simulink model "three_pole_pi"  (R2025b)
settings: Solver=VariableStepAuto  StartTime=0.0  StopTime=120  RelTol=1e-3
model workspace (MAT data in the model file):
  Ki = 20
  Kp = 250
  b = 50
  m = 1000
  u = 10
values from neighbouring files (symbols this model uses):
  l_eff = 9.8/(omega_n^2)    [Rocky_pendulum_parametization.m]
  omega_n = signal_params.omega_n    [Rocky_pendulum_parametization.m]
undefined symbols (not defined in the file or in its folder): alpha, beta
settings Model: Creator=clee1  LastModifiedBy=ssocol
settings SolverCC: AlgebraicLoopSolver=TrustRegion
settings DebuggingCC: UnconnectedInputMsg=warning  UnconnectedOutputMsg=warning  UnconnectedLineMsg=warning
settings ModelReferenceCC: EnableRefExpFcnMdlSchedulingChecks=on
settings RTWCC: GPUComputeCapability=3.5

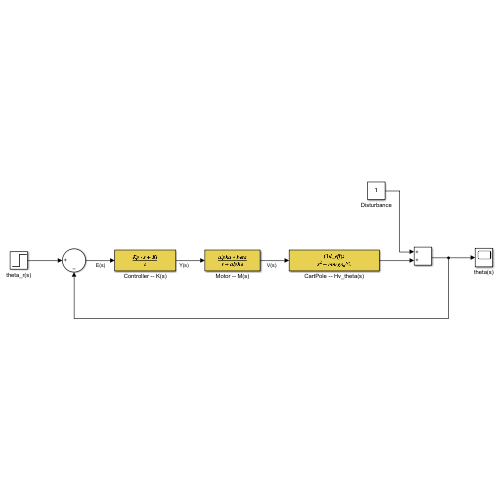
[thumbnail: Simulink's stored preview of the top-level diagram]
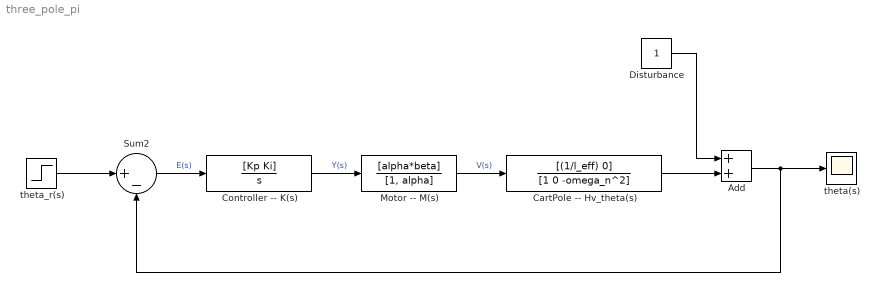
== system three_pole_pi ==
  Add : Sum
  "CartPole -- Hv_theta(s)" : TransferFcn  Numerator=[(1/l_eff) 0]  Denominator=[1 0 -omega_n^2]  ContinuousStateAttributes="\"Controller\""
  "Controller -- K(s)" : TransferFcn  Numerator=[Kp Ki]  Denominator=[1 0]  ContinuousStateAttributes="\"Controller\""
  Disturbance : Constant
  "Motor -- M(s)" : TransferFcn  Numerator=[alpha*beta]  Denominator=[1, alpha]  ContinuousStateAttributes="\"Controller\""
  Sum2 : Sum  Inputs=|+-
  theta(s) : Scope
      settings: ActiveDisplayYMinimum=-5.0682320541648182E+237  ActiveDisplayYMaximum=5.6313689490720195E+236
  theta_r(s) : Step  After=20  SampleTime=0
  wires:
  Sum2/1 -> "Controller -- K(s)"/1  "E(s)"
  "Controller -- K(s)"/1 -> "Motor -- M(s)"/1  "Y(s)"
  "Motor -- M(s)"/1 -> "CartPole -- Hv_theta(s)"/1  "V(s)"
  "CartPole -- Hv_theta(s)"/1 -> Add/2
  theta_r(s)/1 -> Sum2/1
  Add/1 -> Sum2/2, theta(s)/1
  Disturbance/1 -> Add/1
